simulink library "PI_Controller_UL"  (R2019a)
settings: Solver=VariableStepAuto  StartTime=0.0  StopTime=10.0  RelTol=1e-3
undefined symbols (not defined in the file): CTRL
settings Model: Creator=John Jr  LastModifiedBy=John Jr

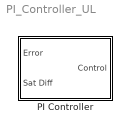
== system PI_Controller_UL ==
  PI Controller : Subsystem  mask{kp=CTRL.Kp, ki=CTRL.Ki}
      mask prompts: kp "Proportional gain"; ki "Integral gain"
      mask DialogControl DescGroupVar Prompt: PI Controller
      mask DialogControl DescTextVar Prompt: This block models a PI controller with anti-windup.
      mask DialogControl Control2 Prompt: Controller Parameters:
      mask Display:
      | patch([0 1 1 0], [0 0 1 1],[.8 1 1])
      | 
      | port_label('input',1,'\fontname{Cambria Math}Error','texmode','on')
      | port_label('input',2,'\fontname{Cambria Math}Sat Diff','texmode','on')
      | 
      | port_label('output',1,'\fontname{Cambria Math}Control','texmode','on')

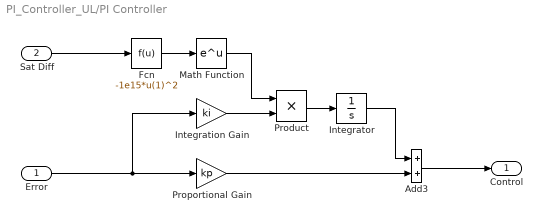
== system PI_Controller_UL/PI Controller ==
  Error : Inport
  Sat Diff : Inport  Port=2
  Add3 : Sum
  Fcn : Fcn  Expr=-1e15*u(1)^2
  Integration Gain : Gain  Gain=ki
  Integrator : Integrator
  Math Function : Math  SaturateOnIntegerOverflow=on
  Product : Product
  Proportional Gain : Gain  Gain=kp
  Control : Outport
  wires:
  Add3/1 -> Control/1
  Fcn/1 -> Math Function/1
  Error/1 -> Integration Gain/1, Proportional Gain/1
  Sat Diff/1 -> Fcn/1
  Math Function/1 -> Product/1
  Proportional Gain/1 -> Add3/2
  Product/1 -> Integrator/1
  Integrator/1 -> Add3/1
  Integration Gain/1 -> Product/2
